simulink model "PID_impedanz_control"  (R2019b)
settings: Solver=FixedStepAuto  StartTime=0.0  StopTime=inf  FixedStep=0.01  RelTol=1e-3
values from neighbouring files (symbols this model uses):
  Ts = 0.01    [RW_LQR_Observer_START.m]    (also in RW_PID_impedanz_START.m; main_start.m)
  Var = 7.5924    [RW_LQR_Observer_START.m]    (also in RW_PID_impedanz_START.m; main_start.m)
libraries: simulink x1, sldrtlib x1
settings Model: EnablePacing=on  Creator=mandl  LastModifiedBy=mandl
settings SolverCC: AlgebraicLoopSolver=LineSearch

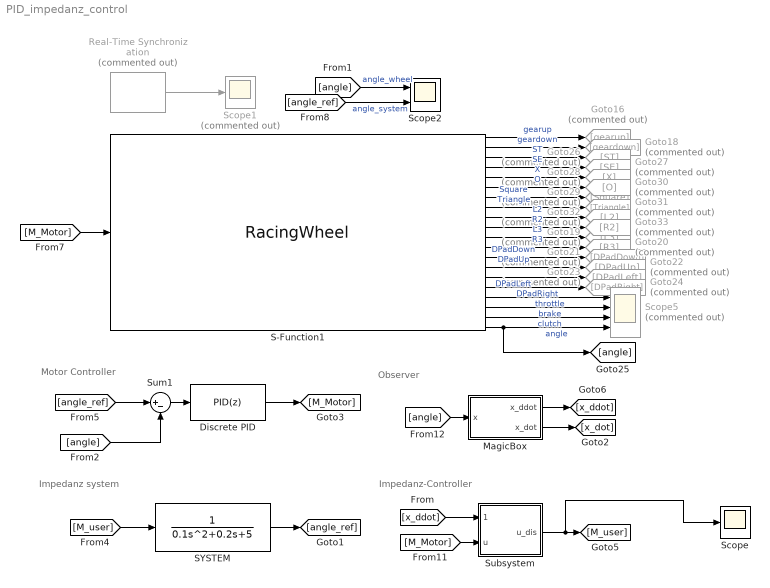
== system PID_impedanz_control ==
  note: Impedanz-Controller
  note: Observer
  note: Impedanz system
  note: Motor Controller
  Discrete PID : simulink/Continuous/PID Controller  Controller=PID  Form=Parallel  TimeDomain=Discrete-time  SampleTime=0.01  IntegratorMethod=Forward Euler  FilterMethod=Forward Euler  ControllerParametersSource=internal  P=5  I=5  D=1  UseFilter=on  N=50  TunerSelectOption=Transfer Function Based (PID Tuner App)  InitialConditionSource=internal  InitialConditionForIntegrator=0  InitialConditionForFilter=0  DifferentiatorICPrevScaledInput=0  ExternalReset=none  TrackingMode=off  Kt=1  LimitOutput=on  UpperSaturationLimit=1  LowerSaturationLimit=-1  LinearizeAsGain=off  AntiWindupMode=clamping  Kb=1  POutMin=[]  POutMax=[]  IOutMin=[]  IOutMax=[]  DOutMin=[]  DOutMax=[]  NOutMin=[]  NOutMax=[]  SumOutMin=[]  SumOutMax=[]  SaturationOutMin=[]  SaturationOutMax=[]  PParamMin=[]  PParamMax=[]  IParamMin=[]  IParamMax=[]  DParamMin=[]  DParamMax=[]  NParamMin=[]  NParamMax=[]  KbParamMin=[]  KbParamMax=[]  KtParamMin=[]  KtParamMax=[]  KbOutMin=[]  KbOutMax=[]  KtOutMin=[]  KtOutMax=[]  IntegratorOutMin=[]  IntegratorOutMax=[]  FilterOutMin=[]  FilterOutMax=[]  SumI1OutMin=[]  SumI1OutMax=[]  SumI2OutMin=[]  SumI2OutMax=[]  SumI3OutMin=[]  SumI3OutMax=[]  SumI4OutMin=[]  SumI4OutMax=[]  SumDOutMin=[]  SumDOutMax=[]  DifferentiatorOutMin=[]  DifferentiatorOutMax=[]  FilterDiffOutCoefMin=[]  FilterDiffOutCoefMax=[]  ReciprocalOutMin=[]  ReciprocalOutMax=[]  SumDenOutMin=[]  SumDenOutMax=[]  SumNumOutMin=[]  SumNumOutMax=[]  DivideOutMin=[]  DivideOutMax=[]  IntegratorContinuousStateAttributes=''  IntegratorStateMustResolveToSignalObject=off  IntegratorRTWStateStorageClass=Auto  FilterContinuousStateAttributes=''  FilterStateMustResolveToSignalObject=off  FilterRTWStateStorageClass=Auto  ParallelPVariant=InternalParameters  IdealPVariant=Disabled  IVariant=InternalParameters  DVariant=InternalParameters  IntegratorVariant=Discrete  SatVariant=Enabled  AWVariant=DiscClampingParallel  PCopyVariant=Disabled  TRVariant=Disabled  FdbkBlocksVariant=Forward  IdealPFdbkVariant=Disabled  SatFdbkVariant=Disabled  DerivativeFilterVariant=ForwardEulerFilter  NVariant=InternalParameters  NCopyVariant=Disabled  FilterICVariant=InternalICsFilter  IntegratorICVariant=InternalICs  ExternalResetVariant=Disabled  TRSumVariant=Passthrough  SumFdbkVariant=Disabled  SumVariant=Sum_PID
  Goto16 : Goto  Commented=on  GotoTag=gearup
  Goto18 : Goto  Commented=on  GotoTag=geardown
  Goto19 : Goto  Commented=on  GotoTag=L3
  Goto20 : Goto  Commented=on  GotoTag=R3
  Goto21 : Goto  Commented=on  GotoTag=DPadDown
  Goto22 : Goto  Commented=on  GotoTag=DPadUp
  Goto23 : Goto  Commented=on  GotoTag=DPadLeft
  Goto24 : Goto  Commented=on  GotoTag=DPadRight
  Goto26 : Goto  Commented=on  GotoTag=ST
  Goto27 : Goto  Commented=on  GotoTag=SE
  Goto28 : Goto  Commented=on  GotoTag=X
  Goto29 : Goto  Commented=on  GotoTag=Square
  Goto30 : Goto  Commented=on  GotoTag=O
  Goto31 : Goto  Commented=on  GotoTag=Triangle
  Goto32 : Goto  Commented=on  GotoTag=L2
  Goto33 : Goto  Commented=on  GotoTag=R2
  MagicBox : Subsystem  mask{N_coeff=3}
      mask prompts: N_coeff "Filter Coef"
  Real-Time Synchronization : sldrtlib/Real-Time Synchronization  Commented=on  SampleTime=0.01  MaxMissedTicks=inf  ShowMissedTicks=on  YieldWhenWaiting=off
  S-Function1 : S-Function  FunctionName=RacingWheel  Parameters=Ts_FF  SFunctionModules=RacingWheel_wrapper  SFunctionDeploymentMode=off  EnableBusSupport=off  mask(Racing Wheel with Force Feedback){Ts_FF=0.01}
      mask prompts: Ts_FF "Constant Force-Feedback Sample Time"
      mask help: Interacts with the windows gaming API from UWP. The force feedback effect is constant over the user defined sampling time below.
      mask init:
      | val = [[.9  0.75 0.75 1 1 .9 .9 1]',[1 1 0.75 0.75 .9 .9 1 .9]'];try , sys = get_param(gcb,'SfunBuilderFcnName');if isempty(sys), sys = get_param(gcb,'FunctionName'); end,catch, sys = get_param(gcb,'FunctionName'); end
      mask Display:
      | plot(val(:,1),val(:,2)),disp(sys),
      | image('icon.png'),
      | port_label('input',1,'FF'),
      | port_label('output',1,'gearup'),
      | port_label('output',2,'geardown'),
      | port_label('output',3,'ST'),
      | port_label('output',4,'SE'),
      | port_label('output',5,'X'),
      | port_label('output',6,'O'),
      | port_label('output',7,'Square'),
      | port_label('output',8,'Triangle'),
      | port_label('output',9,'L2'),
      | port_label('output',10,'R2'),
      | port_label('output',11,'L3'),
      | port_label('output',12,'R3'),
      | port_label('output',13,'DPadDown'),
      | port_label('output',14,'DPadUp'),
      | port_label('output',15,'DPadLeft'),
      | port_label('output',16,'DPadRight'),
      | port_label('output',17,'throttle'),
      | port_label('output',18,'brake'),
      | port_label('output',19,'clutch'),
      | port_label('output',20,'angle')
  SYSTEM : TransferFcn  Denominator=[0.1 0.2 5]
  Scope : Scope
  Scope1 : Scope  Commented=on
  Scope2 : Scope  NumInputPorts=2
  Scope5 : Scope  Commented=on  NumInputPorts=4
  Subsystem : Subsystem
  Sum1 : Sum  Inputs=|+-
  wires:
  Real-Time Synchronization/1 -> Scope1/1
  S-Function1/4 -> Goto27/1  "SE"
  S-Function1/17 -> Scope5/1  "throttle"
  S-Function1/5 -> Goto28/1  "X"
  S-Function1/13 -> Goto21/1  "DPadDown"
  S-Function1/8 -> Goto31/1  "Triangle"
  S-Function1/11 -> Goto19/1  "L3"
  S-Function1/10 -> Goto33/1  "R2"
  S-Function1/1 -> Goto16/1  "gearup"
  S-Function1/18 -> Scope5/2  "brake"
  S-Function1/14 -> Goto22/1  "DPadUp"
  S-Function1/3 -> Goto26/1  "ST"
  S-Function1/6 -> Goto30/1  "O"
  S-Function1/7 -> Goto29/1  "Square"
  S-Function1/15 -> Goto23/1  "DPadLeft"
  S-Function1/9 -> Goto32/1  "L2"
  S-Function1/12 -> Goto20/1  "R3"
  S-Function1/2 -> Goto18/1  "geardown"
  S-Function1/19 -> Scope5/3  "clutch"
  S-Function1/16 -> Goto24/1  "DPadRight"
  S-Function1/20 -> Scope5/4, [angle]  "angle"
  [M_Motor] -> S-Function1/1
  [angle] -> Scope2/1  "angle_wheel"
  SYSTEM/1 -> [angle_ref]
  [M_user] -> SYSTEM/1
  Sum1/1 -> Discrete PID/1
  [angle_ref] -> Sum1/1
  [angle] -> Sum1/2
  Discrete PID/1 -> [M_Motor]
  [angle_ref] -> Scope2/2  "angle_system"
  [x_ddot] -> Subsystem/1(x_ddot)
  [M_Motor] -> Subsystem/2(u)
  Subsystem/1(u_dis) -> Scope/1, [M_user]
  [angle] -> MagicBox/1(x)
  MagicBox/1(x_ddot) -> [x_ddot]
  MagicBox/2(x_dot) -> [x_dot]

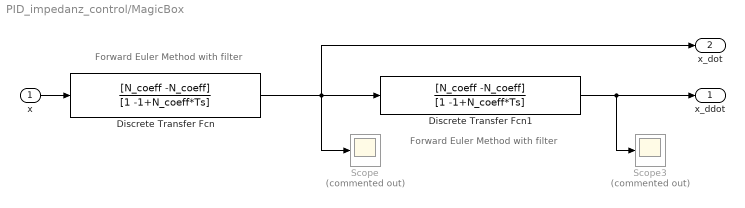
== system PID_impedanz_control/MagicBox ==
  note: Forward Euler Method with filter
  note: Forward Euler Method with filter
  x : Inport
  Discrete Transfer Fcn : DiscreteTransferFcn  Numerator=[N_coeff -N_coeff]  Denominator=[1 -1+N_coeff*Ts]  SampleTime=Ts
  Discrete Transfer Fcn1 : DiscreteTransferFcn  Numerator=[N_coeff -N_coeff]  Denominator=[1 -1+N_coeff*Ts]  SampleTime=Ts
  Scope : Scope  Commented=on
  Scope3 : Scope  Commented=on
  x_ddot : Outport
  x_dot : Outport  Port=2
  wires:
  Discrete Transfer Fcn/1 -> x_dot/1, Scope/1, Discrete Transfer Fcn1/1
  Discrete Transfer Fcn1/1 -> x_ddot/1, Scope3/1
  x/1 -> Discrete Transfer Fcn/1

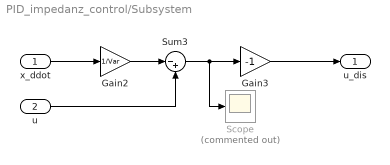
== system PID_impedanz_control/Subsystem ==
  x_ddot : Inport
  u : Inport  Port=2
  Gain2 : Gain  Gain=1/Var
  Gain3 : Gain  Gain=-1
  Scope : Scope  Commented=on
  Sum3 : Sum  Inputs=|-+
  u_dis : Outport
  wires:
  Sum3/1 -> Gain3/1, Scope/1
  Gain2/1 -> Sum3/1
  Gain3/1 -> u_dis/1
  x_ddot/1 -> Gain2/1
  u/1 -> Sum3/2
